simulink model "aeroTestHarness"  (R2024a)
settings: configuration reference "standardSILConfiguraitonParams" (kept outside this file)
undefined symbols (not defined in the file): lbf2N, vehicleParams
settings Model: Creator=jerem  LastModifiedBy=jerem
settings ConfigSetRef: SourceName=standardSILConfiguraitonParams  SourceLocation=Base Workspace

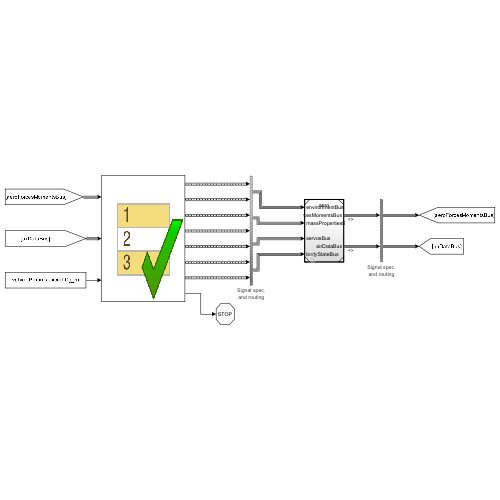
[thumbnail: Simulink's stored preview of the top-level diagram]
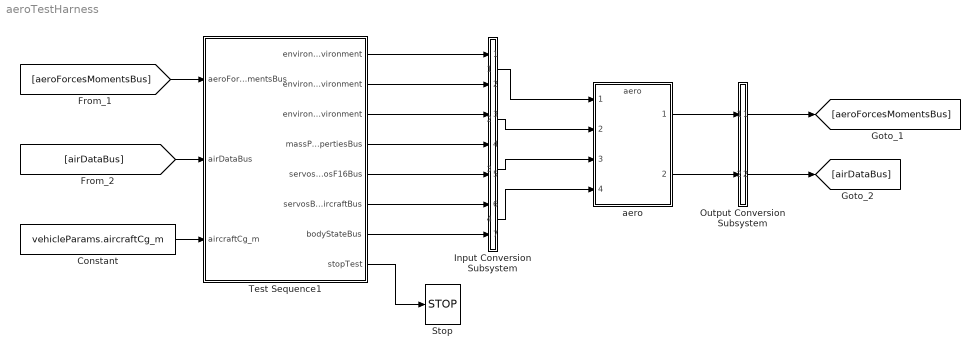
== system aeroTestHarness ==
  Constant : Constant  Value=vehicleParams.aircraftCg_m
  Input Conversion Subsystem : Subsystem  Tag=__SLT_ICS__  Description=|
      | Signal spec.
      | and routing
      settings: AttributesFormatString=%<Description>
  Output Conversion Subsystem : Subsystem  Tag=__SLT_OCS__  Description=|
      | Signal spec.
      | and routing
      mask init:
      | ICDictionary = get_param(bdroot, 'DataDictionary');
      | if isempty(ICDictionary)
      |    ICScope = Simulink.data.BaseWorkspace;
      | else
      |    ICScope = Simulink.data.DataDictionary(ICDictionary);
      | end
      | 
      | IC1 = Simulink.Bus.createMATLABStruct('ComponentForcesMomentsBus', [], [1 1], ICScope);
      | IC2 = Simulink.Bus.createMATLABStruct('AirData', [], [1 1], ICScope);
      settings: AttributesFormatString=%<Description>
  Stop : Stop
  Test Sequence1 : Test Sequence  TreatAsAtomicUnit=on
  aero : ModelReference  ModelNameDialog=aero  SimulationMode=Normal  ModelReferenceVersion=1.297
  wires:
  Test Sequence1/1(environmentBus_EarthEnvironment) -> Input Conversion Subsystem/1(Inport_1)
  Test Sequence1/2(environmentBus_AirEnvironment) -> Input Conversion Subsystem/2(Inport_2)
  Test Sequence1/3(environmentBus_TerrainEnvironment) -> Input Conversion Subsystem/3(Inport_3)
  Test Sequence1/4(massPropertiesBus) -> Input Conversion Subsystem/4(Inport_4)
  Test Sequence1/5(servosBus_ServosF16Bus) -> Input Conversion Subsystem/5(Inport_5)
  Test Sequence1/6(servosBus_ServosCustomAircraftBus) -> Input Conversion Subsystem/6(Inport_6)
  Test Sequence1/7(bodyStateBus) -> Input Conversion Subsystem/7(Inport_7)
  [aeroForcesMomentsBus] -> Test Sequence1/1(aeroForcesMomentsBus)
  [airDataBus] -> Test Sequence1/2(airDataBus)
  Output Conversion Subsystem/1(Outport_1) -> [aeroForcesMomentsBus]
  Output Conversion Subsystem/2(Outport_2) -> [airDataBus]
  Input Conversion Subsystem/1(Outport_1) -> aero/1
  Input Conversion Subsystem/2(Outport_2) -> aero/2
  Input Conversion Subsystem/3(Outport_3) -> aero/3
  Input Conversion Subsystem/4(Outport_4) -> aero/4
  aero/1 -> Output Conversion Subsystem/1(Inport_1)
  aero/2 -> Output Conversion Subsystem/2(Inport_2)
  Test Sequence1/8(stopTest) -> Stop/1
  Constant/1 -> Test Sequence1/3(aircraftCg_m)

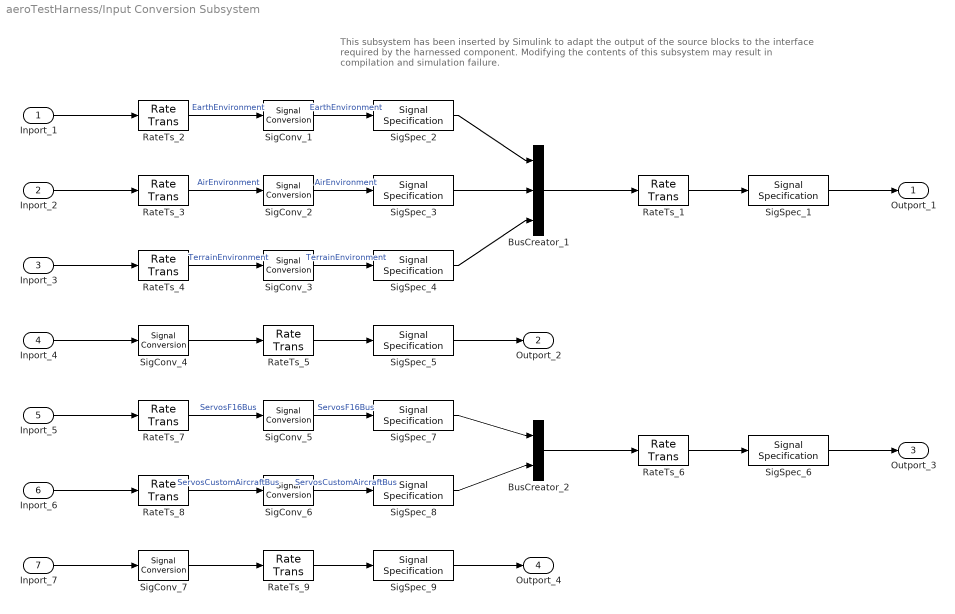
== system aeroTestHarness/Input Conversion Subsystem ==
  note: This subsystem has been inserted by Simulink to adapt the output of the source blocks to the interface required by the harnessed component.
      |  Modifying the contents of this subsystem may result in compilation and simulation failure.
  Inport_1 : Inport
  Inport_2 : Inport  Port=2
  Inport_3 : Inport  Port=3
  Inport_4 : Inport  Port=4
  Inport_5 : Inport  Port=5
  Inport_6 : Inport  Port=6
  Inport_7 : Inport  Port=7
  BusCreator_1 : BusCreator  Inputs=3  OutDataTypeStr=Bus: EnvironmentBus
  BusCreator_2 : BusCreator  Inputs=2  OutDataTypeStr=Bus: ServosBus
  RateTs_{1..9} (9 alike) : RateTransition  OutPortSampleTime=0.004
  SigConv_{1..3,5..6} (5 alike) : SignalConversion  ConversionOutput=Nonvirtual bus  OverrideOpt=off
  SigConv_4 : SignalConversion  ConversionOutput=Virtual bus  OverrideOpt=off
  SigConv_7 : SignalConversion  ConversionOutput=Virtual bus  OverrideOpt=off
  SigSpec_1 : SignalSpecification  OutDataTypeStr=Bus: EnvironmentBus  SampleTime=0.004
  SigSpec_2 : SignalSpecification  OutDataTypeStr=Bus: EarthEnvironmentBus  Dimensions=[1]  SampleTime=0.004  BusOutputAsStruct=on
  SigSpec_3 : SignalSpecification  OutDataTypeStr=Bus: AirEnvironmentBus  Dimensions=[1]  SampleTime=0.004  BusOutputAsStruct=on
  SigSpec_4 : SignalSpecification  OutDataTypeStr=Bus: TerrainEnvironmentBus  Dimensions=[1]  SampleTime=0.004  BusOutputAsStruct=on
  SigSpec_5 : SignalSpecification  OutDataTypeStr=Bus: MassPropertiesBus  SampleTime=0.004
  SigSpec_6 : SignalSpecification  OutDataTypeStr=Bus: ServosBus  SampleTime=0.004
  SigSpec_7 : SignalSpecification  OutDataTypeStr=Bus: ServosF16Bus  Dimensions=[1]  SampleTime=0.004  BusOutputAsStruct=on
  SigSpec_8 : SignalSpecification  OutDataTypeStr=Bus: ServosCustomAircraftBus  Dimensions=[1]  SampleTime=0.004  BusOutputAsStruct=on
  SigSpec_9 : SignalSpecification  OutDataTypeStr=Bus: BodyStateBus  SampleTime=0.004
  Outport_1 : Outport
  Outport_2 : Outport  Port=2
  Outport_3 : Outport  Port=3
  Outport_4 : Outport  Port=4
  wires:
  SigSpec_1/1 -> Outport_1/1
  RateTs_1/1 -> SigSpec_1/1
  BusCreator_1/1 -> RateTs_1/1
  SigSpec_2/1 -> BusCreator_1/1
  SigConv_1/1 -> SigSpec_2/1  "EarthEnvironment"
  RateTs_2/1 -> SigConv_1/1  "EarthEnvironment"
  Inport_1/1 -> RateTs_2/1
  SigSpec_3/1 -> BusCreator_1/2
  SigConv_2/1 -> SigSpec_3/1  "AirEnvironment"
  RateTs_3/1 -> SigConv_2/1  "AirEnvironment"
  Inport_2/1 -> RateTs_3/1
  SigSpec_4/1 -> BusCreator_1/3
  SigConv_3/1 -> SigSpec_4/1  "TerrainEnvironment"
  RateTs_4/1 -> SigConv_3/1  "TerrainEnvironment"
  Inport_3/1 -> RateTs_4/1
  SigSpec_5/1 -> Outport_2/1
  RateTs_5/1 -> SigSpec_5/1
  SigConv_4/1 -> RateTs_5/1
  Inport_4/1 -> SigConv_4/1
  SigSpec_6/1 -> Outport_3/1
  RateTs_6/1 -> SigSpec_6/1
  BusCreator_2/1 -> RateTs_6/1
  SigSpec_7/1 -> BusCreator_2/1
  SigConv_5/1 -> SigSpec_7/1  "ServosF16Bus"
  RateTs_7/1 -> SigConv_5/1  "ServosF16Bus"
  Inport_5/1 -> RateTs_7/1
  SigSpec_8/1 -> BusCreator_2/2
  SigConv_6/1 -> SigSpec_8/1  "ServosCustomAircraftBus"
  RateTs_8/1 -> SigConv_6/1  "ServosCustomAircraftBus"
  Inport_6/1 -> RateTs_8/1
  SigSpec_9/1 -> Outport_4/1
  RateTs_9/1 -> SigSpec_9/1
  SigConv_7/1 -> RateTs_9/1
  Inport_7/1 -> SigConv_7/1

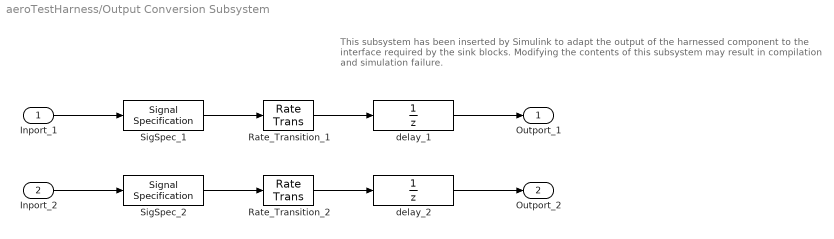
== system aeroTestHarness/Output Conversion Subsystem ==
  note: This subsystem has been inserted by Simulink to adapt the output of the harnessed component to the interface required by the sink blocks.
      |  Modifying the contents of this subsystem may result in compilation and simulation failure.
  Inport_1 : Inport
  Inport_2 : Inport  Port=2
  Rate_Transition_1 : RateTransition  OutPortSampleTimeOpt=Inherit
  Rate_Transition_2 : RateTransition  OutPortSampleTimeOpt=Inherit
  SigSpec_1 : SignalSpecification  OutDataTypeStr=Bus: ComponentForcesMomentsBus  Dimensions=[1]  SampleTime=0.004
  SigSpec_2 : SignalSpecification  OutDataTypeStr=Bus: AirData  Dimensions=[1]  SampleTime=0.004
  delay_1 : UnitDelay  InitialCondition=IC1  SampleTime=-1
  delay_2 : UnitDelay  InitialCondition=IC2  SampleTime=-1
  Outport_1 : Outport
  Outport_2 : Outport  Port=2
  wires:
  Inport_1/1 -> SigSpec_1/1
  SigSpec_1/1 -> Rate_Transition_1/1
  Rate_Transition_1/1 -> delay_1/1
  delay_1/1 -> Outport_1/1
  Inport_2/1 -> SigSpec_2/1
  SigSpec_2/1 -> Rate_Transition_2/1
  Rate_Transition_2/1 -> delay_2/1
  delay_2/1 -> Outport_2/1

== stateflow chart aeroTestHarness/Test Sequence1 ==
  state Scenario_1
    state Initialize
      %% Initialize data outputs.
      environmentBus_EarthEnvironment.gravityScalar_mps2 = 0;
      environmentBus_EarthEnvironment.worldMagneticFieldInNED_nT = zeros(3,1);
      environmentBus_AirEnvironment.airTemperature_K = 0;
      environmentBus_AirEnvironment.airPressure_Pa = 0;
      environmentBus_AirEnvironment.airDensity_kgpm3 = 1.225;
      environmentBus_AirEnvironment.windSpeedInNED_mps = zeros(3,1);
      environmentBus_AirEnvironment.speedOfSound_mps = 0;
      environmentBus_AirEnvironment.windsAloftInNED_mps = zeros(3,1);
      environmentBus_AirEnvironment.gustInNED_mps = zeros(3,1);
      environmentBus_AirEnvironment.turbulenceInNED_mps = zeros(3,1);
      environmentBus_TerrainEnvironment.terrainHeightInNED_m = 0;
      massPropertiesBus.aircraftMass_kg = 0;
      massPropertiesBus.aircraftCg_m = aircraftCg_m;
      massPropertiesBus.aircraftInertiaInBody_kgm2 = zeros(3,3);
      massPropertiesBus.fuelLevelFraction = 0;
      servosBus_ServosF16Bus.posAileron_rad = 0;
      servosBus_ServosF16Bus.posRudder_rad = 0;
      servosBus_ServosF16Bus.posElevator_rad = 0;
      servosBus_ServosCustomAircraftBus.posControlSurfaceOne_rad = 0;
      servosBus_ServosCustomAircraftBus.posControlSurfaceTwo_rad = 0;
      bodyStateBus.aircraftVelInNED_mps = zeros(3,1);
      bodyStateBus.aircraftPosInNED_m = zeros(3,1);
      bodyStateBus.aircraftEulerAngles_rad = zeros(3,1);
      bodyStateBus.aircraftVelInBody_mps = zeros(3,1);
      bodyStateBus.aircraftAngVelInBody_radps = zeros(3,1);
      bodyStateBus.aircraftAngAccelInBody_radps2 = zeros(3,1);
      bodyStateBus.aircraftAccelInBody_mps2 = zeros(3,1);
      bodyStateBus.DCM_be = zeros(3,3);
      stopTest = false;
    state verifyZeroOutputs
      verify(isClose(aeroForcesMomentsBus.forcesInBody_N(1),0))
      verify(isClose(aeroForcesMomentsBus.forcesInBody_N(2),0))
      verify(isClose(aeroForcesMomentsBus.forcesInBody_N(3),0))
      verify(isClose(aeroForcesMomentsBus.momentsInBody_Nm(1),0))
      verify(isClose(aeroForcesMomentsBus.momentsInBody_Nm(2),0))
      verify(isClose(aeroForcesMomentsBus.momentsInBody_Nm(3),0))
      verify(isClose(airDataBus.airspeedInBody_mps(1),0))
      verify(isClose(airDataBus.airspeedInBody_mps(2),0))
      verify(isClose(airDataBus.airspeedInBody_mps(3),0))
      verify(isClose(airDataBus.alpha_rad,0))
      verify(isClose(airDataBus.beta_rad,0))
    state inputAirspeed
      bodyStateBus.aircraftVelInBody_mps(1) = 257; % Cruise for an F16
    state verifyAirspeed
      verify(aeroForcesMomentsBus.forcesInBody_N(1) < 0)
      verify(isClose(aeroForcesMomentsBus.forcesInBody_N(2),0))
      verify(aeroForcesMomentsBus.forcesInBody_N(3) < -20500 * lbf2N) % Must be generating a force greater than vehicle weight
      verify(isClose(aeroForcesMomentsBus.momentsInBody_Nm(1),0))
      verify(aeroForcesMomentsBus.momentsInBody_Nm(2) < 0) % Should be generating a nose down moment
      verify(isClose(aeroForcesMomentsBus.momentsInBody_Nm(3),0))
      verify(isClose(airDataBus.airspeedInBody_mps(2),0))
      verify(isClose(airDataBus.airspeedInBody_mps(3),0))
      verify(isClose(airDataBus.alpha_rad,0))
      verify(isClose(airDataBus.beta_rad,0))
      cruiseZForce = aeroForcesMomentsBus.forcesInBody_N(3);
      cruiseYMoment = aeroForcesMomentsBus.momentsInBody_Nm(2);
    state addElevator
      servosBus_ServosF16Bus.posElevator_rad = deg2rad(-5);
    state verifyElevatorDeflection
      verify(isClose(aeroForcesMomentsBus.forcesInBody_N(2),0))
      verify(aeroForcesMomentsBus.forcesInBody_N(3) > cruiseZForce)
      verify(isClose(aeroForcesMomentsBus.momentsInBody_Nm(1),0))
      verify(aeroForcesMomentsBus.momentsInBody_Nm(2) > cruiseYMoment)
      verify(isClose(aeroForcesMomentsBus.momentsInBody_Nm(3),0))
      verify(isClose(airDataBus.airspeedInBody_mps(2),0))
      verify(isClose(airDataBus.airspeedInBody_mps(3),0))
      verify(isClose(airDataBus.alpha_rad,0))
      verify(isClose(airDataBus.beta_rad,0))
    state removeElevator
      servosBus_ServosF16Bus.posElevator_rad = 0;
    state addRudder
      servosBus_ServosF16Bus.posRudder_rad = deg2rad(10);
    state verifyRudder
      verify(aeroForcesMomentsBus.forcesInBody_N(2) > 0 )
      verify(aeroForcesMomentsBus.forcesInBody_N(3) < 0)
      verify(aeroForcesMomentsBus.momentsInBody_Nm(1) > 0)
      verify(aeroForcesMomentsBus.momentsInBody_Nm(2) < 0) % Should be generating a nose down moment
      verify(aeroForcesMomentsBus.momentsInBody_Nm(3) < 0 )
      verify(isClose(airDataBus.airspeedInBody_mps(2),0))
      verify(isClose(airDataBus.airspeedInBody_mps(3),0))
      verify(isClose(airDataBus.alpha_rad,0))
      verify(isClose(airDataBus.beta_rad,0))
    state removeRudder
      servosBus_ServosF16Bus.posRudder_rad = deg2rad(0);
    state addAileron
      servosBus_ServosF16Bus.posAileron_rad = deg2rad(5);
    state verifyAileron
      verify(aeroForcesMomentsBus.momentsInBody_Nm(1) < 0) % Should create a negative moment
      verify(isClose(aeroForcesMomentsBus.momentsInBody_Nm(2),cruiseYMoment)) % Should equal value that was at cruise
      verify(aeroForcesMomentsBus.momentsInBody_Nm(3) < 0) % In real life I don't think this would be negative. It's negative here because beta and alpha aren't fed back
      verify(isClose(airDataBus.alpha_rad,0))
      verify(isClose(airDataBus.beta_rad,0))
    state EndTest
      stopTest = true;
    (default) -> Initialize
    Initialize -> verifyZeroOutputs : [
        | after(2,sec)
        | ]
    verifyZeroOutputs -> inputAirspeed : [
        | after(1,sec)
        | ]
    inputAirspeed -> verifyAirspeed : [
        | after(5,sec)
        | ]
    verifyAirspeed -> addElevator : [
        | after(2,sec)
        | ]
    addElevator -> verifyElevatorDeflection : [
        | after(2,sec)
        | ]
    verifyElevatorDeflection -> removeElevator : [
        | after(1,sec)
        | ]
    removeElevator -> addRudder : [
        | after(1,sec)
        | ]
    addRudder -> verifyRudder : [
        | after(2,sec)
        | ]
    verifyRudder -> removeRudder : [
        | after(1,sec)
        | ]
    removeRudder -> addAileron : [
        | after(1,sec)
        | ]
    addAileron -> verifyAileron : [
        | after(3,sec)
        | ]
    verifyAileron -> EndTest : [
        | after(1,sec)
        | ]
  (default) -> Scenario_1 : {assert(Active_Scenario_Index == 1,'The value of Scenario Parameter ''Active_Scenario_Index'' is not valid. Use the index of the scenario to specify it.')}
  data: aeroForcesMomentsBus input Bus: ComponentForcesMomentsBus size=[1]; airDataBus input Bus: AirData size=[1]; environmentBus_EarthEnvironment output Bus: EarthEnvironmentBus size=[1]; environmentBus_AirEnvironment output Bus: AirEnvironmentBus size=[1]; environmentBus_TerrainEnvironment output Bus: TerrainEnvironmentBus size=[1]; massPropertiesBus output Bus: MassPropertiesBus size=[1]; servosBus_ServosF16Bus output Bus: ServosF16Bus size=[1]; servosBus_ServosCustomAircraftBus output Bus: ServosCustomAircraftBus size=[1]; bodyStateBus output Bus: BodyStateBus size=[1]; stopTest output; Active_Scenario_Index parameter =1; lbf2N parameter; cruiseZForce local; cruiseYMoment local; aircraftCg_m input
